simulink model "sst"  (R2025a)
settings: Solver=ode1be  StartTime=0.0  StopTime=simlength  FixedStep=tc  MaxStep=ts_sim
values from neighbouring files (symbols this model uses):
  Adrso = eye(2) + Arso*ts_inv    [design_model.m]
  alpha = 35    [design_model.m]
  C1 = 0.5    [design_model.m]
  Crso = [1 0]    [design_model.m]
  DThs_init = 0    [design_model.m]
  E0 = 3.485    [design_model.m]
  E1 = 0.2156    [design_model.m]
  E2 = 0    [design_model.m]
  E3 = 0    [design_model.m]
  E_1 = -1.031    [design_model.m]
  Elog = -0.05    [design_model.m]
  fPWM_DAB = fPWM_INV    (= 35000)    [design_model.m]
  fPWM_INV = 35e3    (= 35000)    [design_model.m]
  freq = 50    [design_model.m]
  I_FS = Iout_ac_rms_nom * sqrt(2) * margin_factor    [design_model.m]
  ki_i_dab = 18    [design_model.m]
  ki_pll = 3140    [design_model.m]
  ki_v_dab = 45    [design_model.m]
  kp_i_dab = 2    [design_model.m]
  kp_pll = 314    [design_model.m]
  kp_v_dab = 8    [design_model.m]
  Ldrso = acker(Adrso',Crso',polesdrso)'    [design_model.m]
  M = 125    [design_model.m]
  number_of_cells = 30    [design_model.m]
  Q = 1000    [design_model.m]
  q1Kalman = ts_inv^2    (= 8.16326530612e-10)    [design_model.m]
  q2Kalman = ts_inv^1    (= 2.85714285714e-05)    [design_model.m]
  q3Kalman = 0    [design_model.m]
  R0 = 0.0035    [design_model.m]
  R1 = 0.0035    [design_model.m]
  rKalman = 1    [design_model.m]
  Tambient = 40    [design_model.m]
  tc = ts_inv/200    (= 1.42857142857e-07)    [design_model.m]
  ts_afe = ts_inv    (= 2.85714285714e-05)    [design_model.m]
  ts_dab = tPWM_DAB*2    (= 5.71428571429e-05)    [design_model.m]
  ts_inv = tPWM_INV    (= 2.85714285714e-05)    [design_model.m]
  V_FS = Vout_dc_nom * margin_factor    (= 500)    [design_model.m]
  weigth = 0.6/6    (= 0.1)    [design_model.m]
undefined symbols (not defined in the file or in its folder): Aresd, Bresd, Cresd, dead_time_DAB, dead_time_INV, iph_grid_pu_ref, ki_afe, kp_afe, LFu1_AFE, n_modules, omega_grid_nom, RLFu1_AFE, ts_battery, tsample, V_phase_normalization_factor, Vdab2_dc_nom
libraries: fl_lib x280, nesl_utility x188, ee_lib x41, cstblocks x4, single_phase_transformer_lib x2, lithium_ion_cell_lib x1, simulink x1
(part 12 of 12)

== matlab function sst/dab_modA/dab_ctrl/modulator1/PWM generator 3/MATLAB Function ==
  data: t input; y output; phase input; period input
function y = trgo(t,phase,period)
x = sin(2*pi/period*t - phase - pi/2);
y = asin(x);

== matlab function sst/dab_modA/dab_ctrl/modulator1/PWM generator 4/MATLAB Function ==
  data: t input; y output; phase input; period input
function y = trgo(t,phase,period)
x = sin(2*pi/period*t - phase - pi/2);
y = asin(x);

== matlab function sst/inverter_modA/single_phase_pll/double_integrator_observer/bounder1 ==
  data: u input; y output
function y = bounder(u)
    
    y = -pi + mod(u+3*pi,2*pi);
   
end

== matlab function sst/inverter_modA/single_phase_pll/double_integrator_observer/bounder2 ==
  data: u input; y output
function y = bounder(u)
    
    y = -pi + mod(u+3*pi,2*pi);
   
end

== matlab function sst/inverter_modA/single_phase_pll/xieta2alphabeta ==
  data: xi input; alpha output; eta input; gamma input; beta output
function [alpha,beta] = xieta2alphabeta(xi,eta,gamma)
    alpha  = xi*cos(gamma) - eta*sin(gamma);
    beta = xi*sin(gamma) + eta*cos(gamma);
end

== matlab function sst/line_source/phase_gen/bounder1 ==
  data: u input; y output
function y = bounder(u)
    
    y = -pi + mod(u+3*pi,2*pi);
end

== matlab function sst/dab_modB/dab_ctrl/modulator1/PWM generator 1/MATLAB Function ==
  data: t input; y output; phase input; period input
function y = trgo(t,phase,period)
x = sin(2*pi/period*t - phase - pi/2);
y = asin(x);

== matlab function sst/dab_modB/dab_ctrl/modulator1/PWM generator 2/MATLAB Function ==
  data: t input; y output; phase input; period input
function y = trgo(t,phase,period)
x = sin(2*pi/period*t - phase - pi/2);
y = asin(x);

== matlab function sst/dab_modB/dab_ctrl/modulator1/PWM generator 3/MATLAB Function ==
  data: t input; y output; phase input; period input
function y = trgo(t,phase,period)
x = sin(2*pi/period*t - phase - pi/2);
y = asin(x);

== matlab function sst/dab_modB/dab_ctrl/modulator1/PWM generator 4/MATLAB Function ==
  data: t input; y output; phase input; period input
function y = trgo(t,phase,period)
x = sin(2*pi/period*t - phase - pi/2);
y = asin(x);

== matlab function sst/inverter_modB/single phase inverter control/pwm/PWM generator 1/MATLAB Function ==
  data: t input; y output; phase input; period input
function y = trgo(t,phase,period)
x = sin(2*pi/period*t - phase - pi/2);
y = asin(x);

== matlab function sst/inverter_modB/single phase inverter control/pwm/PWM generator 2/MATLAB Function ==
  data: t input; y output; phase input; period input
function y = trgo(t,phase,period)
x = sin(2*pi/period*t - phase - pi/2);
y = asin(x);

== matlab function sst/inverter_modB/single_phase_pll/alphabeta2xieta ==
  data: alpha input; xi output; beta input; gamma input; eta output
function [xi,eta] = alphabeta2xieta(alpha,beta,gamma)
    xi  =  alpha*cos(gamma) + beta*sin(gamma);
    eta = -alpha*sin(gamma) + beta*cos(gamma);
end

== matlab function sst/inverter_modB/single_phase_pll/double_integrator_observer/bounder1 ==
  data: u input; y output
function y = bounder(u)
    
    y = -pi + mod(u+3*pi,2*pi);
   
end

== matlab function sst/inverter_modB/single_phase_pll/double_integrator_observer/bounder2 ==
  data: u input; y output
function y = bounder(u)
    
    y = -pi + mod(u+3*pi,2*pi);
   
end

== matlab function sst/inverter_modB/single_phase_pll/xieta2alphabeta ==
  data: xi input; alpha output; eta input; gamma input; beta output
function [alpha,beta] = xieta2alphabeta(xi,eta,gamma)
    alpha  = xi*cos(gamma) - eta*sin(gamma);
    beta = xi*sin(gamma) + eta*cos(gamma);
end

== matlab function sst/battery/LithiumIonBattery/SOC_estimator/Kalman_observer/kalman_observer_gains ==
  data: i input; ts input; l1 output; z input; q1 input; q2 input; q3 input; r input; Q input; l2 output; l3 output
function [l1,l2,l3] = EKF(i,ts,z,q1,q2,q3,r,Q)

    persistent  p11 p12 p13 p21 p22 p23 p31 p32 p33

    if isempty(p11)
        p11 = q1;
        p12 = 0;
        p13 = 0;
        p21 = 0;
        p22 = q2;
        p23 = 0;
        p31 = 0;
        p32 = 0;
        p33 = q3;
    end
    R = 0.15;
    C = 10;
    M = 125;
    E_1 = -1.031;
    E1 = 0.2156;
    E2 = 0;
    E3 = 0;
    Elog = -0.05;
    alpha = 35;

    a11 = 1;
    a12 = 0;
    a13 = 0;
    a21 = 0;
    a22 = exp(-ts/(R*C));
    a23 = 0;
    a31 = 0;
    a32 = 0;
    a33 = abs(exp(-i*ts/Q));

    c1 = -alpha*E_1*abs(exp(-alpha*z)) + E1 + 2*E2*z + 3*E3*z^2 - Elog/(1-z+ts);
    c2 = -R;
    c3 = M;
    
    p11_pr = a11*(a11*p11 + a12*p21 + a13*p31) + a12*(a11*p12 + a12*p22 + a13*p32) + a13*(a11*p13 + a12*p23 + a13*p33) + q1;

    p12_pr = a21*(a11*p11 + a12*p21 + a13*p31) + a22*(a11*p12 + a12*p22 + a13*p32) + a23*(a11*p13 + a12*p23 + a13*p33);

    p13_pr = a31*(a11*p11 + a12*p21 + a13*p31) + a32*(a11*p12 + a12*p22 + a13*p32) + a33*(a11*p13 + a12*p23 + a13*p33);

    p21_pr = a11*(a21*p11 + a22*p21 + a23*p31) + a12*(a21*p12 + a22*p22 + a23*p32) + a13*(a21*p13 + a22*p23 + a23*p33);

    p22_pr = a21*(a21*p11 + a22*p21 + a23*p31) + a22*(a21*p12 + a22*p22 + a23*p32) + a23*(a21*p13 + a22*p23 + a23*p33) + q2;

    p23_pr = a31*(a21*p11 + a22*p21 + a23*p31) + a32*(a21*p12 + a22*p22 + a23*p32) + a33*(a21*p13 + a22*p23 + a23*p33);

    p31_pr = a11*(a31*p11 + a32*p21 + a33*p31) + a12*(a31*p12 + a32*p22 + a33*p32) + a13*(a31*p13 + a32*p23 + a33*p33);

    p32_pr = a21*(a31*p11 + a32*p21 + a33*p31) + a22*(a31*p12 + a32*p22 + a33*p32) + a23*(a31*p13 + a32*p23 + a33*p33);

    p33_pr = a31*(a31*p11 + a32*p21 + a33*p31) + a32*(a31*p12 + a32*p22 + a33*p32) + a33*(a31*p13 + a32*p23 + a33*p33) + q3;

    den = c1*(c1*p11 + c2*p21 + c3*p31) + c2*(c1*p12 + c2*p22 + c3*p32) + c3*(c1*p13 + c2*p23 + c3*p33) + r;
 
    l1 = (c1*p11 + c2*p12 + c3*p13)/den;
    l2 = (c1*p21 + c2*p22 + c3*p23)/den;
    l3 = (c1*p31 + c2*p32 + c3*p33)/den;
    
    p11 = (1 - c1*l1)*p11_pr - c2*l1*p21_pr - c3*l1*p31_pr;
    
    p12 = (1 - c1*l1)*p12_pr - c2*l1*p22_pr - c3*l1*p32_pr;
    
    p13 = (1 - c1*l1)*p13_pr - c2*l1*p23_pr - c3*l1*p33_pr;
    
    p21 = -c1*l2*p11_pr + (1 - c2*l2)*p21_pr - c3*l2*p31_pr;
    
    p22 = -c1*l2*p12_pr + (1 - c2*l2)*p22_pr - c3*l2*p32_pr;
    
    p23 = -c1*l2*p13_pr + (1 - c2*l2)*p23_pr - c3*l2*p33_pr;
    
    p31 = -c1*l3*p11_pr - c2*l3*p21_pr + (1 - c3*l3)*p31_pr;
    
    p32 = -c1*l3*p12_pr - c2*l3*p22_pr + (1 - c3*l3)*p32_pr;
    
    p33 = -c1*l3*p13_pr - c2*l3*p23_pr + (1 - c3*l3)*p33_pr;
end

== matlab function sst/inverter_modA/single_phase_pll/alphabeta2xieta ==
  data: alpha input; xi output; beta input; gamma input; eta output
function [xi,eta] = alphabeta2xieta(alpha,beta,gamma)
    xi  =  alpha*cos(gamma) + beta*sin(gamma);
    eta = -alpha*sin(gamma) + beta*cos(gamma);
end

== matlab function sst/battery/LithiumIonBattery/SOC_estimator/Kalman_observer/lithium-ion battery model ==
  data: i input; SOC output; u output; ts input; Q input; l1 input; l2 input; l3 input; vout input; x output; R0 input; R input; C input; E_1 input; E0 input; E1 input; E2 input; E3 input; Elog input; alpha input; N input; M input
function [SOC, u, x] = lithium_ion_battery(i,ts,Q,l1,l2,l3,vout, R0, R,C, E_1, E0, E1, E2, E3, Elog, alpha, N, M)

    persistent z_po ir_po h_po vout_hat

    if isempty(z_po)
        ir_po = 0;
        h_po = 0;
        z_po = 0.35;        
    end      
        z_pr = z_po - ts/Q*i ;
    
        ir_pr = exp(-ts/(R*C))*ir_po + (1-exp(-ts/(R*C)))*i;

        h_pr = exp(-abs(i)*ts/Q)*h_po - (1-exp(-abs(i)*ts/Q))*sign(i);
        
        OCV = E_1*exp(-z_pr*alpha) + E0 + E1*z_pr + E2*z_pr^2 + E3*z_pr^3 + Elog*log(abs(1-z_pr+ts));
        
        vout_hat = OCV*N + M*h_pr - R*ir_pr - R0*i;
        
        z_po = z_pr + l1*(vout - vout_hat);
        ir_po = ir_pr + l2*(vout - vout_hat);
        h_po = h_pr + l3*(vout - vout_hat);
        u = vout_hat;
        
        x = [z_po; ir_po; h_po];

    SOC = z_po;
end
